simulink model "modele_lineaire"  (R2021a)
settings: Solver=VariableStepAuto  StartTime=0.0  StopTime=tfin  RelTol=1e-11
values from neighbouring files (symbols this model uses):
  A = [zeros(3,3),       eye(3),   zeros(3,2),   zeros(3,2),   zeros(3,3) ... (first row only)    [linearisation.m]    (also in main_lineaire.m)
  Axeq = 0    [main_lineaire.m]    (also in main_lineaire_joey.m)
  Ayeq = 0    [main_lineaire.m]    (also in main_lineaire_joey.m)
  B = [zeros(3,3) ... (first row only)    [linearisation.m]    (also in main_lineaire.m)
  C = [    TDEF', zeros(3,3),  zeros(3,4), zeros(3,3) ... (first row only)    [linearisation.m]    (also in main_lineaire.m)
  D = zeros(7,3)    [linearisation.m]    (also in main_lineaire.m)
  V_eq = RR*ik    [constantes_lineaire.m]    (also in main_lineaire.m = 4.88592)
  z_eq = Pzeq    (= 0.015)    [main_lineaire.m]    (also in main_lineaire_joey.m)
settings Model: Creator=User  LastModifiedBy=User
settings SolverCC: AlgebraicLoopSolver=LineSearch
settings DebuggingCC: SignalInfNanChecking=error

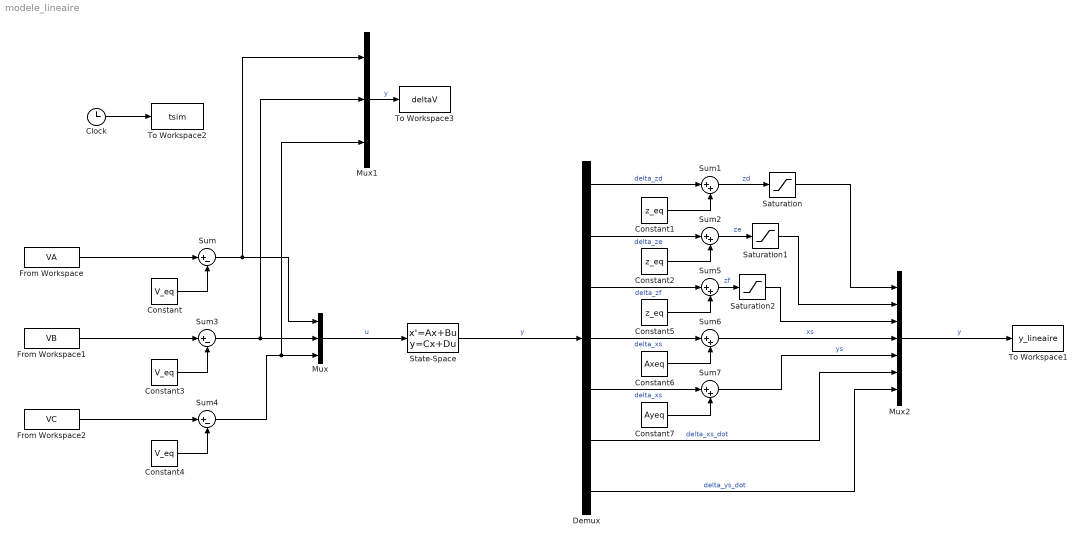
== system modele_lineaire ==
  Clock : Clock
  Constant : Constant  Value=V_eq
  Constant1 : Constant  Value=z_eq
  Constant2 : Constant  Value=z_eq
  Constant3 : Constant  Value=V_eq
  Constant4 : Constant  Value=V_eq
  Constant5 : Constant  Value=z_eq
  Constant6 : Constant  Value=Axeq
  Constant7 : Constant  Value=Ayeq
  Demux : Demux  Outputs=7
  From Workspace : FromWorkspace  VariableName=VA
  From Workspace1 : FromWorkspace  VariableName=VB
  From Workspace2 : FromWorkspace  VariableName=VC
  Mux : Mux  Inputs=3
  Mux1 : Mux  Inputs=3
  Mux2 : Mux  Inputs=7
  Saturation : Saturate  UpperLimit=30/1000  LowerLimit=0
  Saturation1 : Saturate  UpperLimit=30/1000  LowerLimit=0
  Saturation2 : Saturate  UpperLimit=30/1000  LowerLimit=0
  State-Space : StateSpace  A=A  B=B  C=C  D=D  InitialCondition=0
  Sum : Sum  Inputs=|+-
  Sum{1..2,5..7} (5 alike) : Sum  Inputs=|++
  Sum3 : Sum  Inputs=|+-
  Sum4 : Sum  Inputs=|+-
  To Workspace1 : ToWorkspace  VariableName=y_lineaire  SampleTime=-1
  To Workspace2 : ToWorkspace  VariableName=tsim  SampleTime=-1
  To Workspace3 : ToWorkspace  VariableName=deltaV  SampleTime=-1
  wires:
  State-Space/1 -> Demux/1  "y"
  Mux/1 -> State-Space/1  "u"
  From Workspace/1 -> Sum/1
  Clock/1 -> To Workspace2/1
  Constant/1 -> Sum/2
  Sum/1 -> Mux1/1, Mux/1
  From Workspace1/1 -> Sum3/1
  Constant3/1 -> Sum3/2
  From Workspace2/1 -> Sum4/1
  Constant4/1 -> Sum4/2
  Sum4/1 -> Mux1/3, Mux/3
  Sum3/1 -> Mux1/2, Mux/2
  Sum1/1 -> Saturation/1  "zd"
  Sum7/1 -> Mux2/5  "ys"
  Demux/5 -> Sum7/1  "delta_xs"
  Sum6/1 -> Mux2/4  "xs"
  Mux2/1 -> To Workspace1/1  "y"
  Demux/4 -> Sum6/1  "delta_xs"
  Constant6/1 -> Sum6/2
  Sum2/1 -> Saturation1/1  "ze"
  Demux/6 -> Mux2/6  "delta_xs_dot"
  Demux/7 -> Mux2/7  "delta_ys_dot"
  Demux/3 -> Sum5/1  "delta_zf"
  Demux/1 -> Sum1/1  "delta_zd"
  Constant7/1 -> Sum7/2
  Demux/2 -> Sum2/1  "delta_ze"
  Constant1/1 -> Sum1/2
  Constant5/1 -> Sum5/2
  Constant2/1 -> Sum2/2
  Sum5/1 -> Saturation2/1  "zf"
  Mux1/1 -> To Workspace3/1  "y"
  Saturation/1 -> Mux2/1
  Saturation1/1 -> Mux2/2
  Saturation2/1 -> Mux2/3
